simulink model "Pacemaker_Deliverable_2_Final_2023a"  (R2023a)
settings: Solver=FixedStepAuto  StartTime=0.0  StopTime=10.0  FixedStep=1e-3  RelTol=1e-3  EnableMultiTasking=on
undefined symbols (not defined in the file): A0, A1, D0, D1, D10, D11, D12, D13, D2, D3, D5, D6, D8, D9, magnitude, PTA0, PTA1, PTA2, PTB2, PTB3, PTB9, PTC16, PTC17, PTC2, PTC4, PTD0, PTD1, PTD2, PTD3
libraries: frdmk64flib x19, etargetslib x8, simulink x1, dspstat3 x1
settings Model: SimulationMode=external  ExtModeTrigDuration=5  Creator=kelby  LastModifiedBy=kelby
settings OptimizationCC: EnhancedBackFolding=on  PassReuseOutputArgsAs=Individual arguments  ZeroExternalMemoryAtStartup=off  ZeroInternalMemoryAtStartup=off  MaxStackSize=64  OptimizeBlockOrder=speed  DifferentSizesBufferReuse=on  OptimizationCustomize=off  EfficientTunableParamExpr=on
settings DebuggingCC: ParameterTunabilityLossMsg=error
settings HardwareCC: ProdBitPerPointer=32  ProdBitPerSizeT=32  ProdBitPerPtrDiffT=32  ProdLargestAtomicInteger=Long  ProdLargestAtomicFloat=Double  ProdWordSize=32  ProdHWDeviceType=ARM Compatible->ARM Cortex
settings SFSimCC: MATLABDynamicMemAlloc=off
settings RTWCC: Description=Embedded Coder  SystemTargetFile=ert.tlc  HardwareBoard=NXP FRDM-K64F  TLCOptions="-aInlineSetEventsForThisBaseRateFcn=TLC_FALSE -aSuppressMultiTaskScheduler=TLC_FALSE  -aRateBasedStepFcn=0"  TemplateMakefile=ert_default_tmf  Toolchain=GNU Tools for ARM Embedded Processors
settings CodeAppCC: ForceParamTrailComments=on  IgnoreCustomStorageClasses=off  OperatorAnnotations=on  SimulinkDataObjDesc=on  SFDataObjDesc=on  InsertBlockDesc=on
settings ERTTargetCC: ExtMode=on  ExtModeTransport=4  ExtModeMexFile=sendToCommService  ExtModeMexArgs='Pacemaker_Deliverable_2_Merged_AMPARIAN_2023a' 0

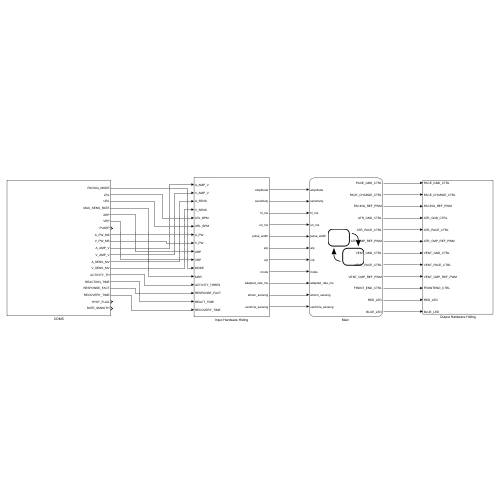
[thumbnail: Simulink's stored preview of the top-level diagram]
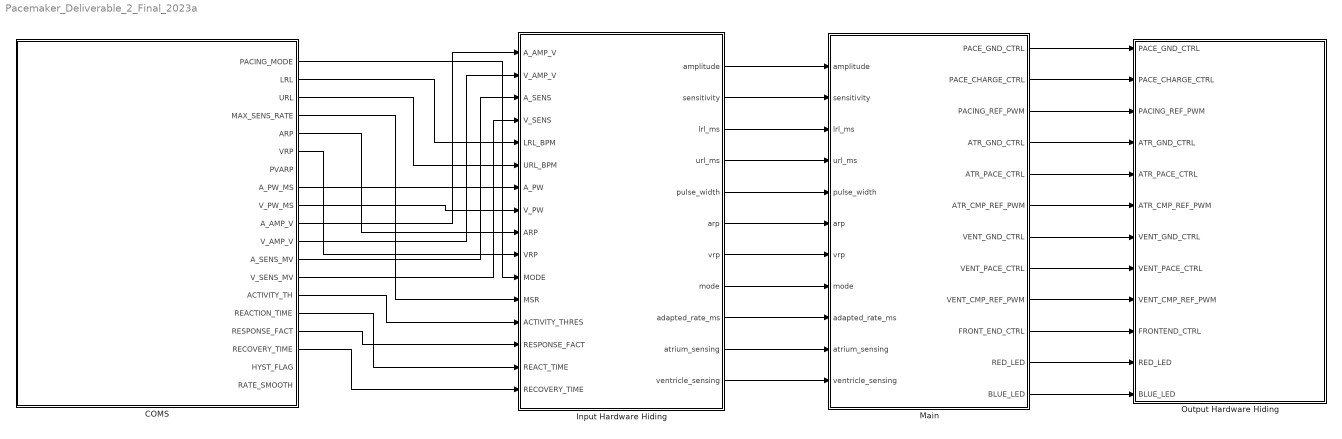
== system Pacemaker_Deliverable_2_Final_2023a ==
  COMS : Subsystem
  Input Hardware Hiding : Subsystem
  "Main " : Stateflow chart  TreatAsAtomicUnit=on
  Output Hardware Hiding : Subsystem
  wires:
  Input Hardware Hiding/1(amplitude) -> "Main "/1(amplitude)
  Input Hardware Hiding/3(lrl_ms) -> "Main "/3(lrl_ms)
  Input Hardware Hiding/4(url_ms) -> "Main "/4(url_ms)
  Input Hardware Hiding/5(pulse_width) -> "Main "/5(pulse_width)
  Input Hardware Hiding/8(mode) -> "Main "/8(mode)
  Input Hardware Hiding/6(arp) -> "Main "/6(arp)
  Input Hardware Hiding/7(vrp) -> "Main "/7(vrp)
  Input Hardware Hiding/2(sensitivity) -> "Main "/2(sensitivity)
  "Main "/4(ATR_GND_CTRL) -> Output Hardware Hiding/4(ATR_GND_CTRL)
  "Main "/5(ATR_PACE_CTRL) -> Output Hardware Hiding/5(ATR_PACE_CTRL)
  "Main "/2(PACE_CHARGE_CTRL) -> Output Hardware Hiding/2(PACE_CHARGE_CTRL)
  "Main "/1(PACE_GND_CTRL) -> Output Hardware Hiding/1(PACE_GND_CTRL)
  "Main "/3(PACING_REF_PWM) -> Output Hardware Hiding/3(PACING_REF_PWM)
  "Main "/7(VENT_GND_CTRL) -> Output Hardware Hiding/7(VENT_GND_CTRL)
  "Main "/8(VENT_PACE_CTRL) -> Output Hardware Hiding/8(VENT_PACE_CTRL)
  "Main "/9(VENT_CMP_REF_PWM) -> Output Hardware Hiding/9(VENT_CMP_REF_PWM)
  "Main "/6(ATR_CMP_REF_PWM) -> Output Hardware Hiding/6(ATR_CMP_REF_PWM)
  "Main "/12(BLUE_LED) -> Output Hardware Hiding/12(BLUE_LED)
  "Main "/11(RED_LED) -> Output Hardware Hiding/11(RED_LED)
  Input Hardware Hiding/10(atrium_sensing) -> "Main "/10(atrium_sensing)
  Input Hardware Hiding/11(ventricle_sensing) -> "Main "/11(ventricle_sensing)
  "Main "/10(FRONT_END_CTRL) -> Output Hardware Hiding/10(FRONTEND_CTRL)
  Input Hardware Hiding/9(adapted_rate_ms) -> "Main "/9(adapted_rate_ms)
  COMS/5(ARP) -> Input Hardware Hiding/9(ARP)
  COMS/3(URL) -> Input Hardware Hiding/6(URL_BPM)
  COMS/4(MAX_SENS_RATE) -> Input Hardware Hiding/12(MSR)
  COMS/6(VRP) -> Input Hardware Hiding/10(VRP)
  COMS/8(A_PW_MS) -> Input Hardware Hiding/7(A_PW)
  COMS/2(LRL) -> Input Hardware Hiding/5(LRL_BPM)
  COMS/10(A_AMP_V) -> Input Hardware Hiding/1(A_AMP_V)
  COMS/1(PACING_MODE) -> Input Hardware Hiding/11(MODE)
  COMS/12(A_SENS_MV) -> Input Hardware Hiding/3(A_SENS)
  COMS/11(V_AMP_V) -> Input Hardware Hiding/2(V_AMP_V)
  COMS/9(V_PW_MS) -> Input Hardware Hiding/8(V_PW)
  COMS/13(V_SENS_MV) -> Input Hardware Hiding/4(V_SENS)
  COMS/14(ACTIVITY_TH) -> Input Hardware Hiding/13(ACTIVITY_THRES)
  COMS/15(REACTION_TIME) -> Input Hardware Hiding/15(REACT_TIME)
  COMS/16(RESPONSE_FACT) -> Input Hardware Hiding/14(RESPONSE_FACT)
  COMS/17(RECOVERY_TIME) -> Input Hardware Hiding/16(RECOVERY_TIME)

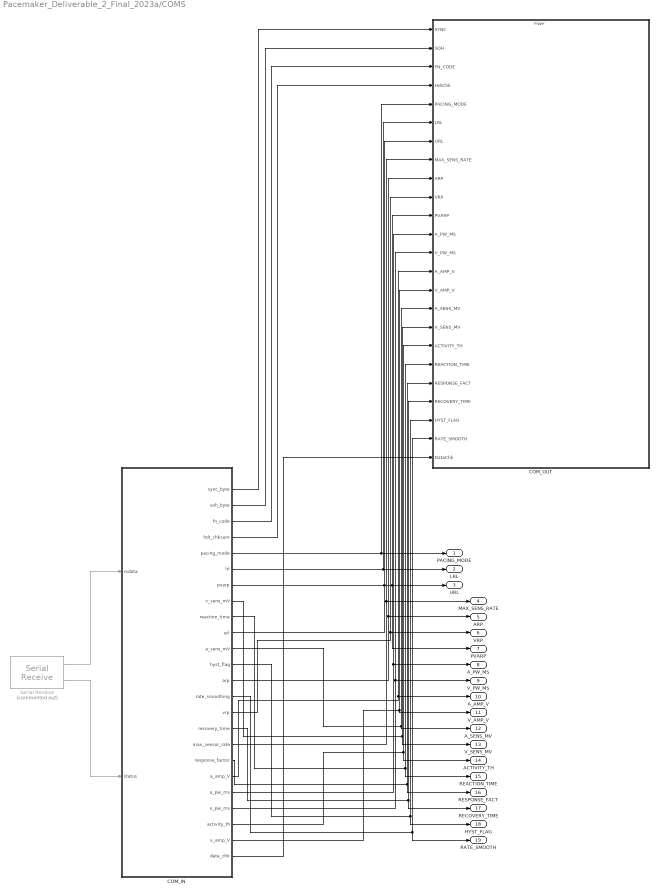
== system Pacemaker_Deliverable_2_Final_2023a/COMS ==
  COM_IN : Stateflow chart  TreatAsAtomicUnit=on
      settings: PortSchema="{\"entries\":[{\"content\":{\"sides\":[{\"content\":{\"connectorIds\":[\"In1\",\"In2\"]},\"type\":\"ConnectorPlacement.EquallySpacedRectSide\",\"uuid\":\"7f42586a-66dd-4cb7-bdec-24e2c61c98c8\"},{\"content\":{\"connectorIds\":[\"Out1\",\"Out2\",\"Out3\",\"Out4\",\"Out5\",\"Out6\",\"Out11\",\"Out17\",\"Out19\",\"Out7\",\"Out16\",\"Out22\",\"Out9\",\"Out23\",\"Out10\",\"Out21\",\"Out8\",\"Out20\",\"Out14\",\"Out12\",\"Out13\",\"Out18\",\"Out15\",\"Out24\"],\"side\":\"RIGHT\"},\"type\":\"ConnectorPlacement.EquallySpacedRectSide\",\"uuid\":\"364e71ac-c1c2-4196-b90e-e30a9c442d8a\"},{\"content\":{\"side\":\"TOP\"},\"type\":\"ConnectorPlacement.EquallySpacedRectSide\",\"uuid\":\"97d98e62-eeec-4242-a861-5e3f19f454fd\"}]},\"type\":\"ConnectorPlacement.EquallySpacedConnector\",\"uuid\":\"1e165215-d51d-43cd-b857-e5e828e79fc4\"}],\"packageUris\":[\"http://schema.mathworks.com/mf0/Connector/R2020b\"],\"version\":\"1.0\"}"
  COM_OUT : Subsystem
  Serial Receive : frdmk64flib/Serial Receive  Commented=on  SCIModule=0  Baudrate=uint32(9600)  Parity=None  StopBits=1  HardwareFlowControl=None  ByteOrder=LittleEndian  DataType=uint8  DataLength=35  BlockingMode=off  OutputStatus=on  SampleTime=-1
  PACING_MODE : Outport
  LRL : Outport  Port=2
  URL : Outport  Port=3
  MAX_SENS_RATE : Outport  Port=4
  ARP : Outport  Port=5
  VRP : Outport  Port=6
  PVARP : Outport  Port=7
  A_PW_MS : Outport  Port=8
  V_PW_MS : Outport  Port=9
  A_AMP_V : Outport  Port=10
  V_AMP_V : Outport  Port=11
  A_SENS_MV : Outport  Port=12
  V_SENS_MV : Outport  Port=13
  ACTIVITY_TH : Outport  Port=14
  REACTION_TIME : Outport  Port=15
  RESPONSE_FACT : Outport  Port=16
  RECOVERY_TIME : Outport  Port=17
  HYST_FLAG : Outport  Port=18
  RATE_SMOOTH : Outport  Port=19
  wires:
  Serial Receive/1 -> COM_IN/1(rxdata)
  Serial Receive/2 -> COM_IN/2(status)
  COM_IN/5(pacing_mode) -> PACING_MODE/1, COM_OUT/5(PACING_MODE)
  COM_IN/6(lrl) -> LRL/1, COM_OUT/6(LRL)
  COM_IN/7(url) -> COM_OUT/7(URL), URL/1
  COM_IN/8(max_sensor_rate) -> MAX_SENS_RATE/1, COM_OUT/8(MAX_SENS_RATE)
  COM_IN/9(arp) -> ARP/1, COM_OUT/9(ARP)
  COM_IN/10(vrp) -> VRP/1, COM_OUT/10(VRP)
  COM_IN/11(pvarp) -> PVARP/1, COM_OUT/11(PVARP)
  COM_IN/12(a_pw_ms) -> A_PW_MS/1, COM_OUT/12(A_PW_MS)
  COM_IN/13(v_pw_ms) -> COM_OUT/13(V_PW_MS), V_PW_MS/1
  COM_IN/14(a_amp_V) -> A_AMP_V/1, COM_OUT/14(A_AMP_V)
  COM_IN/15(v_amp_V) -> V_AMP_V/1, COM_OUT/15("V_AMP_V ")
  COM_IN/16(a_sens_mV) -> A_SENS_MV/1, COM_OUT/16(A_SENS_MV)
  COM_IN/17(v_sens_mV) -> V_SENS_MV/1, COM_OUT/17(V_SENS_MV)
  COM_IN/18(activity_th) -> ACTIVITY_TH/1, COM_OUT/18(ACTIVITY_TH)
  COM_IN/19(reaction_time) -> REACTION_TIME/1, COM_OUT/19(REACTION_TIME)
  COM_IN/20(response_factor) -> RESPONSE_FACT/1, COM_OUT/20(RESPONSE_FACT)
  COM_IN/21(recovery_time) -> RECOVERY_TIME/1, COM_OUT/21(RECOVERY_TIME)
  COM_IN/22(hyst_flag) -> HYST_FLAG/1, COM_OUT/22(HYST_FLAG)
  COM_IN/23(rate_smoothing) -> RATE_SMOOTH/1, COM_OUT/23(RATE_SMOOTH)
  COM_IN/1(sync_byte) -> COM_OUT/1(SYNC)
  COM_IN/2(soh_byte) -> COM_OUT/2(SOH)
  COM_IN/3(fn_code) -> COM_OUT/3(FN_CODE)
  COM_IN/4(hdr_chksum) -> COM_OUT/4(HdrChk)
  COM_IN/24(data_chk) -> COM_OUT/24(DataChk)

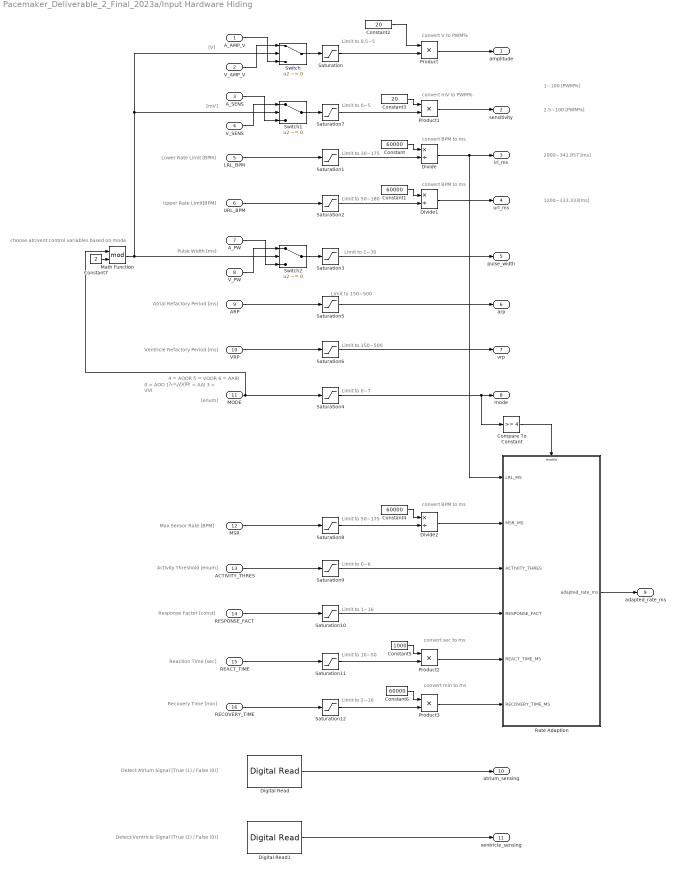
== system Pacemaker_Deliverable_2_Final_2023a/Input Hardware Hiding ==
  note: choose atr/vent control variables based on mode
  note: 0 = AOO
      | 1 = VOO
      | 2 = AAI
      | 3 = VVI
  note: Detect Atrium Signal [True (1) / False (0)]
  note: Limit to 0.5~5
  note: convert BPM to ms
  note: Ventricle Refactory Period [ms]
  note: Atrial Refactory Period [ms]
  note: convert BPM to ms
  note: Limit to 30~175
  note: Limit to 50~180
  note: Limit to 1~30
  note: Limit to 0~7
  note: Limit to 150~500
  note: Limit to 150~500
  note: Limit to 0~5
  note: convert V to PWM%
  note: convert mV to PWM%
  note: [mV]
  note: 2.5~100 [PWM%]
  note: 1~100 [PWM%]
  note: Lower Rate Limit [BPM]
  note: Upper Rate Limit[BPM]
  note: 2000~342.857 [ms]
  note: 1200~333.333[ms]
  note: Pulse Width [ms]
  note: [enum]
  note: [V]
  note: Detect Ventricle Signal [True (1) / False (0)]
  note: convert min to ms
  note: Max Sensor Rate [BPM]
  note: Activity Threshold [enum]
  note: Limit to 1~16
  note: Reaction Time [sec]
  note: Response Factor [const]
  note: Limit to 50~175
  note: Limit to 10~50
  note: Limit to 0~6
  note: Limit to 2~16
  note: Recovery Time [min]
  note: convert sec to ms
  note: convert BPM to ms
  note: 4 = AOOR
      | 5 = VOOR
      | 6 = AAIR
      | 7 = VVIR
  A_AMP_V : Inport
  V_AMP_V : Inport  Port=2
  A_SENS : Inport  Port=3
  V_SENS : Inport  Port=4
  LRL_BPM : Inport  Port=5
  URL_BPM : Inport  Port=6
  A_PW : Inport  Port=7
  V_PW : Inport  Port=8
  ARP : Inport  Port=9
  VRP : Inport  Port=10
  MODE : Inport  Port=11  OutDataTypeStr=uint8
  MSR : Inport  Port=12
  ACTIVITY_THRES : Inport  Port=13
  RESPONSE_FACT : Inport  Port=14
  REACT_TIME : Inport  Port=15
  RECOVERY_TIME : Inport  Port=16
  Compare To Constant : simulink/Logic and Bit Operations/Compare To Constant  relop=>=  const=4  OutDataTypeStr=boolean
  Constant{,1,4,6} (4 alike) : Constant  Value=60000
  Constant2 : Constant  Value=20
  Constant3 : Constant  Value=20
  Constant5 : Constant  Value=1000
  Constant7 : Constant  Value=2  OutDataTypeStr=uint8
  Digital Read : frdmk64flib/Digital Read  Whichpin=PTC16 (D0)  SampleTime=-1
  Digital Read1 : frdmk64flib/Digital Read  Whichpin=PTC17 (D1)  SampleTime=-1
  Divide : Product  Inputs=*/
  Divide1 : Product  Inputs=*/
  Divide2 : Product  Inputs=*/
  Math Function : Math  Operator=mod
  Product{,1..3} (4 alike) : Product
  Rate Adaption : Subsystem  TreatAsAtomicUnit=on
  Saturation : Saturate  UpperLimit=5  LowerLimit=0.5
  Saturation1 : Saturate  UpperLimit=175  LowerLimit=30
  Saturation10 : Saturate  UpperLimit=16  LowerLimit=1
  Saturation11 : Saturate  UpperLimit=50  LowerLimit=10
  Saturation12 : Saturate  UpperLimit=16  LowerLimit=2
  Saturation2 : Saturate  UpperLimit=180  LowerLimit=50
  Saturation3 : Saturate  UpperLimit=30  LowerLimit=1
  Saturation4 : Saturate  UpperLimit=7  LowerLimit=0
  Saturation5 : Saturate  UpperLimit=500  LowerLimit=150
  Saturation6 : Saturate  UpperLimit=500  LowerLimit=150
  Saturation7 : Saturate  UpperLimit=5  LowerLimit=0
  Saturation8 : Saturate  UpperLimit=175  LowerLimit=50
  Saturation9 : Saturate  UpperLimit=6  LowerLimit=0
  Switch : Switch  Criteria=u2 ~= 0  SaturateOnIntegerOverflow=off  InputSameDT=off
  Switch1 : Switch  Criteria=u2 ~= 0  SaturateOnIntegerOverflow=off  InputSameDT=off
  Switch2 : Switch  Criteria=u2 ~= 0  SaturateOnIntegerOverflow=off  InputSameDT=off
  amplitude : Outport
  sensitivity : Outport  Port=2
  lrl_ms : Outport  Port=3
  url_ms : Outport  Port=4
  pulse_width : Outport  Port=5
  arp : Outport  Port=6
  vrp : Outport  Port=7
  mode : Outport  Port=8
  adapted_rate_ms : Outport  Port=9
  atrium_sensing : Outport  Port=10
  ventricle_sensing : Outport  Port=11
  wires:
  LRL_BPM/1 -> Saturation1/1
  Saturation1/1 -> Divide/2
  Constant/1 -> Divide/1
  URL_BPM/1 -> Saturation2/1
  Saturation3/1 -> pulse_width/1
  MODE/1 -> Saturation4/1, Math Function/1
  Saturation4/1 -> Compare To Constant/1, mode/1
  ARP/1 -> Saturation5/1
  Saturation5/1 -> arp/1
  Saturation6/1 -> vrp/1
  VRP/1 -> Saturation6/1
  Digital Read1/1 -> ventricle_sensing/1
  Digital Read/1 -> atrium_sensing/1
  Constant1/1 -> Divide1/1
  Saturation2/1 -> Divide1/2
  Divide1/1 -> url_ms/1
  Saturation/1 -> Product/2
  Constant2/1 -> Product/1
  Product/1 -> amplitude/1
  Product1/1 -> sensitivity/1
  Saturation7/1 -> Product1/2
  Constant3/1 -> Product1/1
  Constant4/1 -> Divide2/1
  ACTIVITY_THRES/1 -> Saturation9/1
  REACT_TIME/1 -> Saturation11/1
  RESPONSE_FACT/1 -> Saturation10/1
  Saturation11/1 -> Product2/2
  Saturation12/1 -> Product3/2
  Saturation8/1 -> Divide2/2
  Constant5/1 -> Product2/1
  Constant6/1 -> Product3/1
  Saturation10/1 -> Rate Adaption/4(RESPONSE_FACT)
  Product2/1 -> Rate Adaption/5(REACT_TIME_MS)
  Product3/1 -> Rate Adaption/6(RECOVERY_TIME_MS)
  RECOVERY_TIME/1 -> Saturation12/1
  Saturation9/1 -> Rate Adaption/3(ACTIVITY_THRES)
  MSR/1 -> Saturation8/1
  Divide2/1 -> Rate Adaption/2(MSR_MS)
  Divide/1 -> Rate Adaption/1(LRL_MS), lrl_ms/1
  Compare To Constant/1 -> Rate Adaption/Enable
  Rate Adaption/1(adapted_rate_ms) -> adapted_rate_ms/1
  Switch/1 -> Saturation/1
  A_AMP_V/1 -> Switch/3
  V_AMP_V/1 -> Switch/1
  Math Function/1 -> Switch/2, Switch1/2, Switch2/2
  Constant7/1 -> Math Function/2
  V_SENS/1 -> Switch1/1
  A_SENS/1 -> Switch1/3
  Switch1/1 -> Saturation7/1
  Switch2/1 -> Saturation3/1
  A_PW/1 -> Switch2/3
  V_PW/1 -> Switch2/1

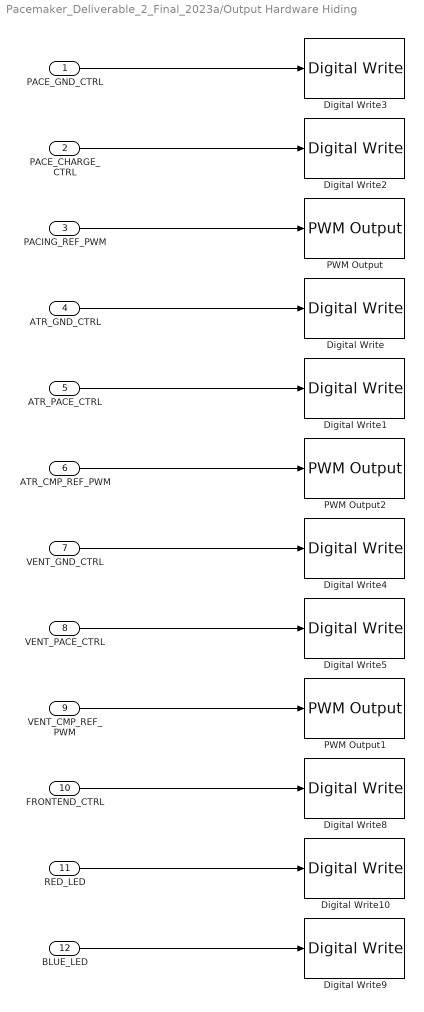
== system Pacemaker_Deliverable_2_Final_2023a/Output Hardware Hiding ==
  PACE_GND_CTRL : Inport
  PACE_CHARGE_CTRL : Inport  Port=2
  PACING_REF_PWM : Inport  Port=3
  ATR_GND_CTRL : Inport  Port=4
  ATR_PACE_CTRL : Inport  Port=5
  ATR_CMP_REF_PWM : Inport  Port=6
  VENT_GND_CTRL : Inport  Port=7
  VENT_PACE_CTRL : Inport  Port=8
  VENT_CMP_REF_PWM : Inport  Port=9
  FRONTEND_CTRL : Inport  Port=10
  RED_LED : Inport  Port=11
  BLUE_LED : Inport  Port=12
  Digital Write : frdmk64flib/Digital Write  Whichpin=PTD2 (D11)
  Digital Write1 : frdmk64flib/Digital Write  Whichpin=PTA0 (D8)
  Digital Write10 : frdmk64flib/Digital Write  Whichpin=RED_LED
  Digital Write2 : frdmk64flib/Digital Write  Whichpin=PTB9 (D2)
  Digital Write3 : frdmk64flib/Digital Write  Whichpin=PTD0 (D10)
  Digital Write4 : frdmk64flib/Digital Write  Whichpin=PTD3 (D12)
  Digital Write5 : frdmk64flib/Digital Write  Whichpin=PTC4 (D9)
  Digital Write8 : frdmk64flib/Digital Write  Whichpin=PTD1 (D13)
  Digital Write9 : frdmk64flib/Digital Write  Whichpin=BLUE_LED
  PWM Output : frdmk64flib/PWM Output  Whichpin=PTA2 (D5)  InitialFrequency=2000  InitialDutyCycle=0
  PWM Output1 : frdmk64flib/PWM Output  Whichpin=PTA1 (D3)  InitialFrequency=2000  InitialDutyCycle=0
  PWM Output2 : frdmk64flib/PWM Output  Whichpin=PTC2 (D6)  InitialFrequency=2000  InitialDutyCycle=0
  wires:
  VENT_GND_CTRL/1 -> Digital Write4/1
  PACE_GND_CTRL/1 -> Digital Write3/1
  VENT_PACE_CTRL/1 -> Digital Write5/1
  PACING_REF_PWM/1 -> PWM Output/1
  PACE_CHARGE_CTRL/1 -> Digital Write2/1
  ATR_PACE_CTRL/1 -> Digital Write1/1
  ATR_GND_CTRL/1 -> Digital Write/1
  VENT_CMP_REF_PWM/1 -> PWM Output1/1
  ATR_CMP_REF_PWM/1 -> PWM Output2/1
  BLUE_LED/1 -> Digital Write9/1
  RED_LED/1 -> Digital Write10/1
  FRONTEND_CTRL/1 -> Digital Write8/1

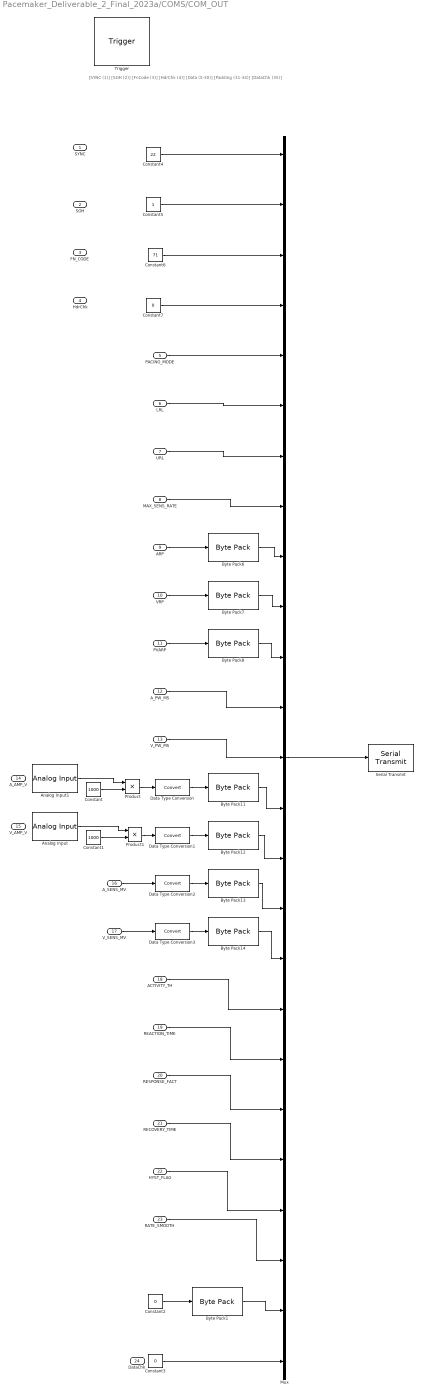
== system Pacemaker_Deliverable_2_Final_2023a/COMS/COM_OUT ==
  note: [SYNC (1)] [SOH (2)] [FnCode (3)] [HdrChk (4)] [Data (5-30)] [Padding (31-34)] [DataChk (35)]
  SYNC : Inport
  SOH : Inport  Port=2
  FN_CODE : Inport  Port=3
  HdrChk : Inport  Port=4
  PACING_MODE : Inport  Port=5
  LRL : Inport  Port=6
  URL : Inport  Port=7
  MAX_SENS_RATE : Inport  Port=8
  ARP : Inport  Port=9
  VRP : Inport  Port=10
  PVARP : Inport  Port=11
  A_PW_MS : Inport  Port=12
  V_PW_MS : Inport  Port=13
  A_AMP_V : Inport  Port=14
  "V_AMP_V " : Inport  Port=15
  A_SENS_MV : Inport  Port=16
  V_SENS_MV : Inport  Port=17
  ACTIVITY_TH : Inport  Port=18
  REACTION_TIME : Inport  Port=19
  RESPONSE_FACT : Inport  Port=20
  RECOVERY_TIME : Inport  Port=21
  HYST_FLAG : Inport  Port=22
  RATE_SMOOTH : Inport  Port=23
  DataChk : Inport  Port=24
  Trigger : TriggerPort  TriggerType=function-call  IsSimulinkFunction=on  FunctionName=send_params  VariantControl=Variant  PortDimensions=1
  Analog Input : frdmk64flib/Analog Input  Whichpin=PTB3 (A1)  SampleTime=-1
  Analog Input1 : frdmk64flib/Analog Input  Whichpin=PTB2 (A0)  SampleTime=-1
  Byte Pack1 : etargetslib/Byte Pack  datatypes={'uint32'}  byteAlign=1
  Byte Pack{6..8,11..14} (7 alike) : etargetslib/Byte Pack  datatypes={'uint16'}  byteAlign=1
  Constant : Constant  Value=1000
  Constant1 : Constant  Value=1000
  Constant2 : Constant  Value=0  OutDataTypeStr=uint32
  Constant3 : Constant  Value=0  OutDataTypeStr=uint8
  Constant4 : Constant  Value=22  OutDataTypeStr=uint8
  Constant5 : Constant  OutDataTypeStr=uint8
  Constant6 : Constant  Value=71  OutDataTypeStr=uint8
  Constant7 : Constant  Value=0  OutDataTypeStr=uint8
  Data Type Conversion{,1..3} (4 alike) : DataTypeConversion  SaturateOnIntegerOverflow=off  RndMeth=Floor
  Mux : Mux  Inputs=25
  Product : Product
  Product1 : Product
  Serial Transmit : frdmk64flib/Serial Transmit  SCIModule=0  Baudrate=uint32(9600)  Parity=None  StopBits=1  HardwareFlowControl=None  ByteOrder=LittleEndian  BlockingMode=on  OutputStatus=off
  wires:
  Mux/1 -> Serial Transmit/1
  ARP/1 -> Byte Pack6/1
  PACING_MODE/1 -> Mux/5
  LRL/1 -> Mux/6
  URL/1 -> Mux/7
  MAX_SENS_RATE/1 -> Mux/8
  Byte Pack6/1 -> Mux/9
  Byte Pack7/1 -> Mux/10
  Byte Pack8/1 -> Mux/11
  A_PW_MS/1 -> Mux/12
  V_PW_MS/1 -> Mux/13
  Byte Pack11/1 -> Mux/14
  Byte Pack12/1 -> Mux/15
  Byte Pack13/1 -> Mux/16
  Byte Pack14/1 -> Mux/17
  ACTIVITY_TH/1 -> Mux/18
  VRP/1 -> Byte Pack7/1
  PVARP/1 -> Byte Pack8/1
  RESPONSE_FACT/1 -> Mux/20
  HYST_FLAG/1 -> Mux/22
  REACTION_TIME/1 -> Mux/19
  RECOVERY_TIME/1 -> Mux/21
  RATE_SMOOTH/1 -> Mux/23
  Constant/1 -> Product/2
  Analog Input1/1 -> Product/1
  Constant1/1 -> Product1/2
  Analog Input/1 -> Product1/1
  Constant2/1 -> Byte Pack1/1
  Byte Pack1/1 -> Mux/24
  Constant3/1 -> Mux/25
  Product/1 -> Data Type Conversion/1
  Data Type Conversion/1 -> Byte Pack11/1
  Product1/1 -> Data Type Conversion1/1
  Data Type Conversion1/1 -> Byte Pack12/1
  A_SENS_MV/1 -> Data Type Conversion2/1
  V_SENS_MV/1 -> Data Type Conversion3/1
  Data Type Conversion2/1 -> Byte Pack13/1
  Data Type Conversion3/1 -> Byte Pack14/1
  Constant7/1 -> Mux/4
  Constant6/1 -> Mux/3
  Constant5/1 -> Mux/2
  Constant4/1 -> Mux/1

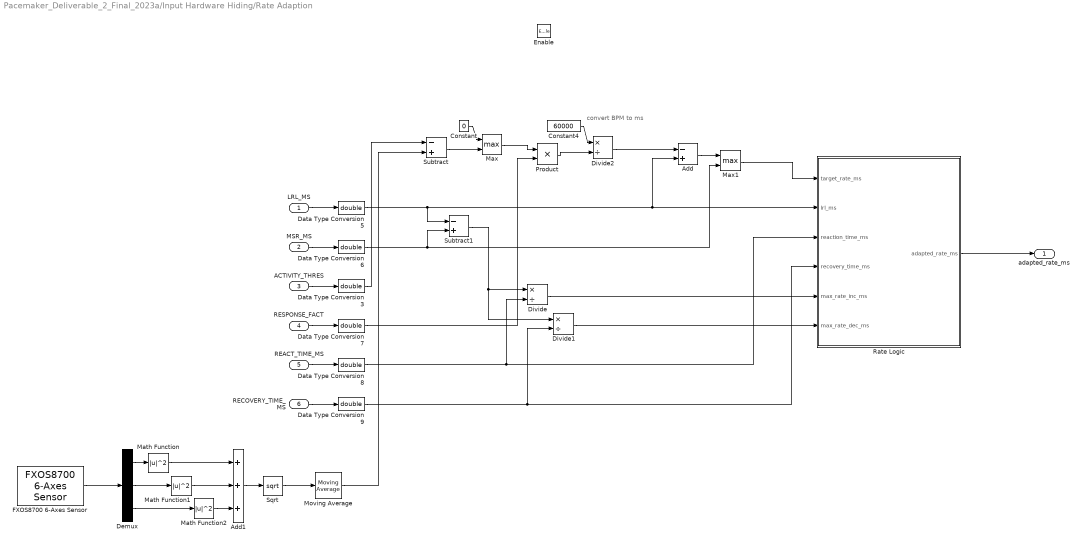
== system Pacemaker_Deliverable_2_Final_2023a/Input Hardware Hiding/Rate Adaption ==
  note: convert BPM to ms
  LRL_MS : Inport
  MSR_MS : Inport  Port=2
  ACTIVITY_THRES : Inport  Port=3
  RESPONSE_FACT : Inport  Port=4
  REACT_TIME_MS : Inport  Port=5
  RECOVERY_TIME_MS : Inport  Port=6
  Enable : EnablePort
  Add : Sum  Inputs=-+
  Add1 : Sum  Inputs=+++
  Constant : Constant  Value=0
  Constant4 : Constant  Value=60000
  Data Type Conversion{3,5..9} (6 alike) : DataTypeConversion  OutDataTypeStr=double  SaturateOnIntegerOverflow=off  RndMeth=Floor
  Demux : Demux  Outputs=3
  Divide : Product  Inputs=*/
  Divide1 : Product  Inputs=*/
  Divide2 : Product  Inputs=*/
  FXOS8700 6-Axes Sensor : frdmk64flib/FXOS8700 6-Axes Sensor  Activesensor=Accelerometer only  ODR=100Hz  HybridODR=400Hz  Accelfullrange=-4g to +4g  SampleTime=-1
  Math Function : Math  Operator=magnitude^2
  Math Function1 : Math  Operator=magnitude^2
  Math Function2 : Math  Operator=magnitude^2
  Max : MinMax  Function=max  Inputs=2
  Max1 : MinMax  Function=max  Inputs=2
  Moving Average : dspstat3/Moving Average  Method=Sliding window  ForgettingFactorPort=off  SpecifyWindowLength=on  WindowLength=100  OverlapLength=99  AllowArbitraryInputLength=off  ForgettingFactor=0.9  SimulateUsing=Code generation
  Product : Product
  Rate Logic : Stateflow chart  TreatAsAtomicUnit=on
  Sqrt : Sqrt
  Subtract : Sum  Inputs=-+
  Subtract1 : Sum  Inputs=-+
  adapted_rate_ms : Outport
  wires:
  Moving Average/1 -> Subtract/2
  Demux/3 -> Math Function2/1
  Add1/1 -> Sqrt/1
  Math Function1/1 -> Add1/2
  Math Function2/1 -> Add1/3
  RECOVERY_TIME_MS/1 -> Data Type Conversion9/1
  MSR_MS/1 -> Data Type Conversion6/1
  Constant4/1 -> Divide2/1
  Subtract1/1 -> Divide/1, Divide1/1
  Math Function/1 -> Add1/1
  Rate Logic/1(adapted_rate_ms) -> adapted_rate_ms/1
  REACT_TIME_MS/1 -> Data Type Conversion8/1
  Add/1 -> Max1/1
  Max/1 -> Product/1
  Subtract/1 -> Max/2
  LRL_MS/1 -> Data Type Conversion5/1
  Demux/2 -> Math Function1/1
  Constant/1 -> Max/1
  Demux/1 -> Math Function/1
  Product/1 -> Divide2/2
  FXOS8700 6-Axes Sensor/1 -> Demux/1
  Sqrt/1 -> Moving Average/1
  RESPONSE_FACT/1 -> Data Type Conversion7/1
  Data Type Conversion5/1 -> Rate Logic/2(lrl_ms), Add/2, Subtract1/1
  Data Type Conversion8/1 -> Rate Logic/3(reaction_time_ms), Divide/2
  Divide1/1 -> Rate Logic/6(max_rate_dec_ms)
  Divide/1 -> Rate Logic/5(max_rate_inc_ms)
  Data Type Conversion9/1 -> Rate Logic/4(recovery_time_ms), Divide1/2
  Max1/1 -> Rate Logic/1(target_rate_ms)
  Data Type Conversion6/1 -> Max1/2, Subtract1/2
  ACTIVITY_THRES/1 -> Data Type Conversion3/1
  Data Type Conversion3/1 -> Subtract/1
  Data Type Conversion7/1 -> Product/2
  Divide2/1 -> Add/1

== stateflow chart Pacemaker_Deliverable_2_Final_2023a/COMS/COM_IN ==
  note: [SYNC (1)] [SOH (2)] [FnCode (3)] [HdrChk (4)] [Data (5-30)] [Padding (31-34)] [DataChk (35)]
  state INITIAL
    entry:
    sync_byte = uint8(0);  % Should be 0x16
    soh_byte = uint8(0);  % Should be 0x01
    fn_code = uint8(0);  % Function code: K_PPARAMS, K_ECHO, etc
    hdr_chksum = uint8(0);
    pacing_mode = uint8(3);
    lrl = uint8(60);
    url = uint8(120);
    max_sensor_rate = uint8(120);
    arp = uint16(250);
    vrp = uint16(320);
    pvarp = uint16(250);
    a_pw_ms = uint8(1);
    v_pw_ms = uint8(1);
    a_amp_raw = uint16(350);
    a_amp_V = 3.5;
    v_amp_raw = uint16(350);
    v_amp_V = 3.5;
    a_sens_raw = uint16(250);
    a_sens_mV = 2.5;
    v_sens_raw = uint16(250);
    v_sens_mV = 2.5;
    activity_th = uint8(3);
    reaction_time = uint8(30);
    response_factor = uint8(8);
    recovery_time = uint8(5);
    hyst_flag = uint8(0);
    rate_smoothing = uint8(0);
    data_chk = uint8(0);  % Data checksum over bytes 5–34
  state SET_PARAM
    entry:
    sync_byte = uint8(rxdata(1));  % Should be 0x16
    soh_byte = uint8(rxdata(2));  % Should be 0x01
    fn_code = uint8(rxdata(3));  % Function code: K_PPARAMS, K_ECHO, etc
    hdr_chksum = uint8(rxdata(4));
    pacing_mode = uint8(rxdata(5));   % Pacing Mode index
    lrl = uint8(rxdata(6));   % Lower Rate Limit (bpm)
    url = uint8(rxdata(7));   % Upper Rate Limit (bpm)
    max_sensor_rate = uint8(rxdata(8));   % Max Sensor Rate (bpm)
    arp = typecast(rxdata(9:10),  'uint16'); % Atrial Refractory Period (ms)
    vrp = typecast(rxdata(11:12), 'uint16'); % Ventricular Refractory Period (ms)
    pvarp = typecast(rxdata(13:14), 'uint16'); % Post Ventricular Atrial Refractory Period (ms)
    a_pw_ms = uint8(rxdata(15));  % Atrial pacing pulse width (ms)
    v_pw_ms = uint8(rxdata(16));  % Ventricular pacing pulse width (ms)
    a_amp_raw = typecast(rxdata(17:18), 'uint16'); % Atrial amplitude, raw = amplitude * 100
    a_amp_V = double(a_amp_raw)  / 100.0;  % Atrial amplitude (V)
    v_amp_raw = typecast(rxdata(19:20), 'uint16'); % Ventricular amplitude, raw = amplitude * 100
    v_amp_V = double(v_amp_raw)  / 100.0;  % Ventricular amplitude (V)
    a_sens_raw = typecast(rxdata(21:22), 'uint16'); % Atrial sensitivity, raw = sensitivity * 100
    a_sens_mV = double(a_sens_raw) / 100.0;  % Atrial sensitivity (mV)
    v_sens_raw = typecast(rxdata(23:24), 'uint16'); % Ventricular sensitivity, raw = sensitivity * 100
    v_sens_mV = double(v_sens_raw) / 100.0;  % Ventricular sensitivity (mV)
    activity_th = uint8(rxdata(25)); % Activity Threshold index
    reaction_time = uint8(rxdata(26)); % Reaction Time (s)
    response_factor = uint8(rxdata(27)); % Response Factor
    recovery_time = uint8(rxdata(28)); % Recovery Time (min)
    hyst_flag = uint8(rxdata(29)); % Hysteresis flag (0 = Off, 1 = On)
    rate_smoothing = uint8(rxdata(30)); % Rate Smoothing index
    data_chk = uint8(rxdata(35));  % Data checksum over bytes 5–34
  state STANDBY
    %Waiting for COM
  state ECHO_PARAM
    entry:
    send_params();
  (default) -> INITIAL
  SET_PARAM -> STANDBY
  INITIAL -> STANDBY
  (junction 10) -> SET_PARAM [order 2] : [rxdata(3) == hex2dec('55')]
  (junction 7) -> STANDBY [order 2]
  STANDBY -> (junction 7) : [status == 0]
  (junction 7) -> (junction 10) [order 1] : [rxdata(1) == hex2dec('16')]
  (junction 10) -> ECHO_PARAM [order 1] : [rxdata(3) == hex2dec('49') || hex2dec('47')]
  ECHO_PARAM -> STANDBY [order 2] : [rxdata(3) == hex2dec('62')]
  ECHO_PARAM -> ECHO_PARAM [order 1] : [after(5,msec)]
  data: sync_byte output; soh_byte output; fn_code output; hdr_chksum output; pacing_mode output; rxdata input uint8; status input uint8; lrl output; url output; max_sensor_rate output; arp output; vrp output; pvarp output; a_pw_ms output uint8; v_pw_ms output; a_amp_V output; v_amp_V output; a_sens_mV output double; v_sens_mV output double; activity_th output; reaction_time output; response_factor output; recovery_time output; hyst_flag output; rate_smoothing output; a_amp_raw local; a_sens_raw local; v_amp_raw local; v_sens_raw local; data_chk output

== stateflow chart Pacemaker_Deliverable_2_Final_2023a/Main  ==
  state AOO
    state AOO_Entry
      entry:
      % all ventricle controls set to 0
      PACING_REF_PWM = amplitude;
      PACE_GND_CTRL = 1;
      VENT_PACE_CTRL = 0;
      VENT_GND_CTRL = 0;
      RED_LED = 1;
      BLUE_LED = 0;
    state AOO_Charging
      entry:
      % charge C22, discharge C21
      PACE_CHARGE_CTRL = 1;
      ATR_PACE_CTRL = 0;
      ATR_GND_CTRL = 1;
    state AOO_Pacing
      entry:
      % pacing atrium
      PACE_CHARGE_CTRL = 0;
      ATR_PACE_CTRL = 1;
      ATR_GND_CTRL = 0;
    note: % total elapse time/cycle = lrl_ms
    (default) -> AOO_Entry
    AOO_Entry -> AOO_Charging
    AOO_Charging -> AOO_Pacing : [after(double(lrl_ms) - double(pulse_width), msec)]
    AOO_Pacing -> AOO_Charging : [after(double(pulse_width), msec)]
  state AOOR
    state AOOR_Entry
      entry:
      % all ventricle controls set to 0
      PACING_REF_PWM = amplitude;
      PACE_GND_CTRL = 1;
      VENT_PACE_CTRL = 0;
      VENT_GND_CTRL = 0;
      RED_LED = 1;
      BLUE_LED = 0;
    state AOOR_Charging
      entry:
      % charge C22, discharge C21
      PACE_CHARGE_CTRL = 1;
      ATR_PACE_CTRL = 0;
      ATR_GND_CTRL = 1;
    state AOOR_Pacing
      entry:
      % pacing atrium
      PACE_CHARGE_CTRL = 0;
      ATR_PACE_CTRL = 1;
      ATR_GND_CTRL = 0;
    note: % total elapse time/cycle = lrl_ms
    (default) -> AOOR_Entry
    AOOR_Entry -> AOOR_Charging
    AOOR_Charging -> AOOR_Pacing : [after(double(adapted_rate_ms) - double(pulse_width), msec)]
    AOOR_Pacing -> AOOR_Charging : [after(double(pulse_width), msec)]
  state VVIR
    state VVIR_Entry
      entry:
      % all atrium controls set to 0
      % ventricle variables set to be same as charging state to be ready for pacing
      PACING_REF_PWM = amplitude;
      VENT_CMP_REF_PWM = sensitivity;
      PACE_CHARGE_CTRL = 1;
      PACE_GND_CTRL = 1;
      ATR_PACE_CTRL = 0;
      ATR_GND_CTRL = 0;
      VENT_PACE_CTRL = 0;
      VENT_GND_CTRL = 1;
      BLUE_LED = 0;
      RED_LED = 0;
      heartbeat_detected = 0;
    state VVIR_Charging
      entry:
      % charge C22, discharge C21
      PACE_CHARGE_CTRL = 1;
      VENT_PACE_CTRL = 0;
      VENT_GND_CTRL = 1;
    state VVIR_Idle
      entry:
      % waiting for heartbeat / time to pace
      BLUE_LED = 0;
    state VVIR_Detected
      entry:
      % heartbeat (ventricle) detected
      heartbeat_detected = 1;
    note: % total elapse time/cycle = lrl_ms
        | (regardless of heartbeat detected or not)
    state VVIR_Pacing
      entry:
      % pacing ventricle
      PACE_CHARGE_CTRL = 0;
      VENT_PACE_CTRL = 1;
      VENT_GND_CTRL = 0;
      BLUE_LED = 1;
      heartbeat_detected = 0;
    (default) -> VVIR_Entry
    VVIR_Entry -> VVIR_Idle
    VVIR_Idle -> VVIR_Detected [order 1] : [ventricle_sensing == 1]
    VVIR_Charging -> VVIR_Idle
    VVIR_Detected -> VVIR_Idle : [after(double(vrp), msec)]
    VVIR_Idle -> VVIR_Pacing [order 2] : [after(double(adapted_rate_ms) - double(pulse_width) - heartbeat_detected * double(vrp), msec)]
    VVIR_Pacing -> VVIR_Charging : [after(double(pulse_width), msec)]
  state Idle
    entry:
    FRONT_END_CTRL = 1;
  state VVI
    state VVI_Entry
      entry:
      % all atrium controls set to 0
      % ventricle variables set to be same as charging state to be ready for pacing
      PACING_REF_PWM = amplitude;
      VENT_CMP_REF_PWM = sensitivity;
      PACE_CHARGE_CTRL = 1;
      PACE_GND_CTRL = 1;
      ATR_PACE_CTRL = 0;
      ATR_GND_CTRL = 0;
      VENT_PACE_CTRL = 0;
      VENT_GND_CTRL = 1;
      BLUE_LED = 0;
      RED_LED = 0;
      heartbeat_detected = 0;
    state VVI_Charging
      entry:
      % charge C22, discharge C21
      PACE_CHARGE_CTRL = 1;
      VENT_PACE_CTRL = 0;
      VENT_GND_CTRL = 1;
    state VVI_Idle
      entry:
      % waiting for heartbeat / time to pace
      BLUE_LED = 0;
    state VVI_Detected
      entry:
      % heartbeat (ventricle) detected
      heartbeat_detected = 1;
    note: % total elapse time/cycle = lrl_ms
        | (regardless of heartbeat detected or not)
    state VVI_Pacing
      entry:
      % pacing ventricle
      PACE_CHARGE_CTRL = 0;
      VENT_PACE_CTRL = 1;
      VENT_GND_CTRL = 0;
      BLUE_LED = 1;
      heartbeat_detected = 0;
    (default) -> VVI_Entry
    VVI_Entry -> VVI_Idle
    VVI_Idle -> VVI_Detected [order 1] : [ventricle_sensing == 1]
    VVI_Charging -> VVI_Idle
    VVI_Detected -> VVI_Idle : [after(double(vrp), msec)]
    VVI_Idle -> VVI_Pacing [order 2] : [after(double(lrl_ms) - double(pulse_width) - heartbeat_detected * double(vrp), msec)]
    VVI_Pacing -> VVI_Charging : [after(double(pulse_width), msec)]
  state VOO
    state VOO_Entry
      entry:
      % all atrium controls set to 0
      PACING_REF_PWM = amplitude;
      PACE_GND_CTRL = 1;
      ATR_PACE_CTRL = 0;
      ATR_GND_CTRL = 0;
      RED_LED = 0;
      BLUE_LED = 1;
    state VOO_Charging
      entry:
      % charge C22, discharge C21
      PACE_CHARGE_CTRL = 1;
      VENT_PACE_CTRL = 0;
      VENT_GND_CTRL = 1;
    state VOO_Pacing
      entry:
      % pacing ventricle
      PACE_CHARGE_CTRL = 0;
      VENT_PACE_CTRL = 1;
      VENT_GND_CTRL = 0;
    note: % total elapse time/cycle = lrl_ms
    (default) -> VOO_Entry
    VOO_Entry -> VOO_Charging
    VOO_Charging -> VOO_Pacing : [after(double(lrl_ms) - double(pulse_width), msec)]
    VOO_Pacing -> VOO_Charging : [after(double(pulse_width), msec)]
  state AAIR
    state AAIR_Entry
      entry:
      % all ventricle controls set to 0
      % atrium variables set to be same as charging state to be ready for pacing
      PACING_REF_PWM = amplitude;
      ATR_CMP_REF_PWM = sensitivity;
      PACE_CHARGE_CTRL = 1;
      PACE_GND_CTRL = 1;
      ATR_PACE_CTRL = 0;
      ATR_GND_CTRL = 1;
      VENT_PACE_CTRL = 0;
      VENT_GND_CTRL = 0;
      BLUE_LED = 0;
      RED_LED = 0;
      heartbeat_detected = 0;
    state AAIR_Charging
      entry:
      % charge C22, discharge C21
      PACE_CHARGE_CTRL = 1;
      ATR_PACE_CTRL = 0;
      ATR_GND_CTRL = 1;
    state AAIR_Idle
      entry:
      % waiting for heartbeat / time to pace
      RED_LED = 0;
    state AAIR_Detected
      entry:
      % heartbeat (atrium) detected
      heartbeat_detected = 1;
    note: % total elapse time/cycle = lrl_ms
        | (regardless of heartbeat detected or not)
    state AAIR_Pacing
      entry:
      % pacing atrium
      PACE_CHARGE_CTRL = 0;
      ATR_PACE_CTRL = 1;
      ATR_GND_CTRL = 0;
      RED_LED = 1;
      heartbeat_detected = 0;
    (default) -> AAIR_Entry
    AAIR_Entry -> AAIR_Idle
    AAIR_Idle -> AAIR_Detected [order 1] : [atrium_sensing == 1]
    AAIR_Charging -> AAIR_Idle
    AAIR_Detected -> AAIR_Idle : [after(double(arp), msec)]
    AAIR_Idle -> AAIR_Pacing [order 2] : [after(double(adapted_rate_ms) - double(pulse_width) - heartbeat_detected * double(arp), msec)]
    AAIR_Pacing -> AAIR_Charging : [after(double(pulse_width), msec)]
  state AAI
    state AAI_Entry
      entry:
      % all ventricle controls set to 0
      % atrium variables set to be same as charging state to be ready for pacing
      PACING_REF_PWM = amplitude;
      ATR_CMP_REF_PWM = sensitivity;
      PACE_CHARGE_CTRL = 1;
      PACE_GND_CTRL = 1;
      ATR_PACE_CTRL = 0;
      ATR_GND_CTRL = 1;
      VENT_PACE_CTRL = 0;
      VENT_GND_CTRL = 0;
      BLUE_LED = 0;
      RED_LED = 0;
      heartbeat_detected = 0;
    state AAI_Charging
      entry:
      % charge C22, discharge C21
      PACE_CHARGE_CTRL = 1;
      ATR_PACE_CTRL = 0;
      ATR_GND_CTRL = 1;
    state AAI_Idle
      entry:
      % waiting for heartbeat / time to pace
      RED_LED = 0;
    state AAI_Detected
      entry:
      % heartbeat (atrium) detected
      heartbeat_detected = 1;
    note: % total elapse time/cycle = lrl_ms
        | (regardless of heartbeat detected or not)
    state AAI_Pacing
      entry:
      % pacing atrium
      PACE_CHARGE_CTRL = 0;
      ATR_PACE_CTRL = 1;
      ATR_GND_CTRL = 0;
      RED_LED = 1;
      heartbeat_detected = 0;
    (default) -> AAI_Entry
    AAI_Entry -> AAI_Idle
    AAI_Idle -> AAI_Detected [order 1] : [atrium_sensing == 1]
    AAI_Charging -> AAI_Idle
    AAI_Detected -> AAI_Idle : [after(double(arp), msec)]
    AAI_Idle -> AAI_Pacing [order 2] : [after(double(lrl_ms) - double(pulse_width) - heartbeat_detected * double(arp), msec)]
    AAI_Pacing -> AAI_Charging : [after(double(pulse_width), msec)]
  state VOOR
    state VOOR_Entry
      entry:
      % all atrium controls set to 0
      PACING_REF_PWM = amplitude;
      PACE_GND_CTRL = 1;
      ATR_PACE_CTRL = 0;
      ATR_GND_CTRL = 0;
      RED_LED = 0;
      BLUE_LED = 1;
    state VOOR_Charging
      entry:
      % charge C22, discharge C21
      PACE_CHARGE_CTRL = 1;
      VENT_PACE_CTRL = 0;
      VENT_GND_CTRL = 1;
    state VOOR_Pacing
      entry:
      % pacing ventricle
      PACE_CHARGE_CTRL = 0;
      VENT_PACE_CTRL = 1;
      VENT_GND_CTRL = 0;
    note: % total elapse time/cycle = lrl_ms
    (default) -> VOOR_Entry
    VOOR_Entry -> VOOR_Charging
    VOOR_Charging -> VOOR_Pacing : [after(double(adapted_rate_ms) - double(pulse_width), msec)]
    VOOR_Pacing -> VOOR_Charging : [after(double(pulse_width), msec)]
  Idle -> AOOR [order 5] : [mode == 4]
  VVIR -> Idle : [mode ~= 7]
  Idle -> VVIR [order 8] : [mode == 7]
  AOO -> Idle : [mode ~= 0]
  Idle -> AOO [order 1] : [mode == 0]
  AOOR -> Idle : [mode ~= 4]
  (default) -> Idle
  VOO -> Idle : [mode ~= 1]
  Idle -> VVI [order 4] : [mode == 3]
  Idle -> VOO [order 2] : [mode == 1]
  VVI -> Idle : [mode ~= 3]
  AAIR -> Idle : [mode ~= 6]
  Idle -> VOOR [order 6] : [mode == 5]
  Idle -> AAIR [order 7] : [mode == 6]
  Idle -> AAI [order 3] : [mode == 2]
  AAI -> Idle : [mode ~= 2]
  VOOR -> Idle : [mode ~= 5]
  data: PACE_GND_CTRL output; PACE_CHARGE_CTRL output; PACING_REF_PWM output; amplitude input; sensitivity input; lrl_ms input; url_ms input; pulse_width input; arp input; vrp input; mode input; adapted_rate_ms input; atrium_sensing input; ventricle_sensing input; ATR_GND_CTRL output; ATR_PACE_CTRL output; ATR_CMP_REF_PWM output; VENT_GND_CTRL output; VENT_PACE_CTRL output; VENT_CMP_REF_PWM output; FRONT_END_CTRL output; RED_LED output; BLUE_LED output; heartbeat_detected local

== stateflow chart Pacemaker_Deliverable_2_Final_2023a/Input Hardware Hiding/Rate Adaption/Rate Logic ==
  state Init
    entry:
    adapted_rate_ms = lrl_ms
  state Idle
  state IncreaseRate
    entry:
    adapted_rate_ms = adapted_rate_ms - max_rate_inc_ms
  state DecreaseRate
    entry:
    adapted_rate_ms = adapted_rate_ms + max_rate_dec_ms
  state WaitReactRecovTime
  state AtTargetRate
    entry:
    adapted_rate_ms = target_rate_ms
  (default) -> Init
  Init -> Idle
  Idle -> Idle [order 2] : [double(adapted_rate_ms) == double(target_rate_ms)]
  Idle -> IncreaseRate [order 1] : [double(adapted_rate_ms) > double(target_rate_ms)]
  Idle -> DecreaseRate [order 3] : [double(adapted_rate_ms) < double(target_rate_ms)]
  DecreaseRate -> AtTargetRate [order 1] : [adapted_rate_ms >= target_rate_ms]
  WaitReactRecovTime -> DecreaseRate [order 3] : [adapted_rate_ms < target_rate_ms && after(recovery_time_ms, msec)]
  DecreaseRate -> WaitReactRecovTime [order 2] : [adapted_rate_ms < target_rate_ms]
  IncreaseRate -> WaitReactRecovTime [order 1] : [adapted_rate_ms > target_rate_ms]
  WaitReactRecovTime -> IncreaseRate [order 1] : [adapted_rate_ms > target_rate_ms && after(reaction_time_ms, msec)]
  IncreaseRate -> AtTargetRate [order 2] : [adapted_rate_ms <= target_rate_ms]
  WaitReactRecovTime -> Idle [order 2] : [adapted_rate_ms == target_rate_ms && after(reaction_time_ms, msec)]
  AtTargetRate -> WaitReactRecovTime
  data: target_rate_ms input; lrl_ms input; reaction_time_ms input; recovery_time_ms input; max_rate_inc_ms input; adapted_rate_ms output; max_rate_dec_ms input
